simulink model "tune"  (R2018a)
settings: Solver=VariableStepAuto  StartTime=0.0  StopTime=10.0  RelTol=1e-3
libraries: simulink x1, simulink_extras x1
settings Model: Creator=rahul  LastModifiedBy=rahul

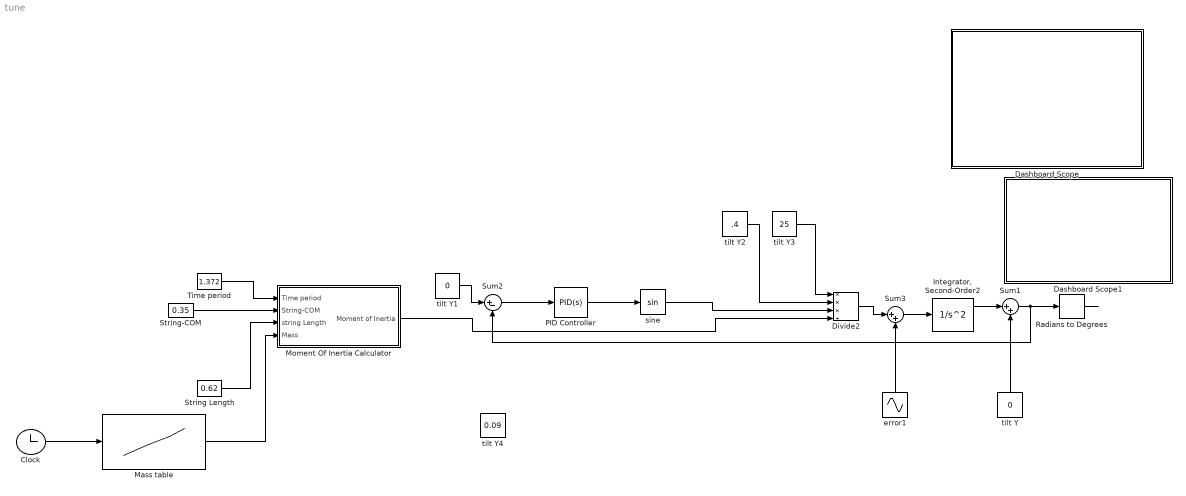
== system tune ==
  Clock : Clock
  Dashboard Scope : Subsystem  DialogController=hmiCreateDDGDialog  IsWebBlock=on  mask(MWDashboardBlock){webBlockId=e338c714-fa8b-4a2a-a1ae-3623556dac48, webBlockType=sdiscope, ShowInitialText=on, HMISrcModelName=tune}
      mask prompts: webBlockId "WebBlock Id"; webBlockType "WebBlock Type"; HMISrcModelName "Source Model"
      mask help: SimulinkHMI:dialogs:HMIScopeDialogDesc
      mask Help: helpview([docroot '/mapfiles/simulink.map'], 'hmi_scope')
      mask Display:
      | if strcmp(get_param(bdroot(gcb),'BlockDiagramType'), 'library')
      |     image([(matlabroot) '/toolbox/simulink/hmi/icons/DashboardScope.png']);
      | end
  Dashboard Scope1 : Subsystem  DialogController=hmiCreateDDGDialog  IsWebBlock=on  mask(MWDashboardBlock){webBlockId=b475c485-489d-4b06-bb0e-a7e4dee8d715, webBlockType=sdiscope, ShowInitialText=on, HMISrcModelName=tune}
      mask prompts: webBlockId "WebBlock Id"; webBlockType "WebBlock Type"; HMISrcModelName "Source Model"
      mask help: SimulinkHMI:dialogs:HMIScopeDialogDesc
      mask Help: helpview([docroot '/mapfiles/simulink.map'], 'hmi_scope')
      mask Display:
      | if strcmp(get_param(bdroot(gcb),'BlockDiagramType'), 'library')
      |     image([(matlabroot) '/toolbox/simulink/hmi/icons/DashboardScope.png']);
      | end
  Divide2 : Product  Inputs=***/
  "Integrator, Second-Order2" : SecondOrderIntegrator
  Mass table : Lookup  InputValues=[0,1]  Table=[0.975,.8]  LookUpMeth=Use Input Nearest  SaturateOnIntegerOverflow=on
  Moment Of Inertia Calculator : Subsystem
  PID Controller : simulink/Continuous/PID Controller  Controller=PID  TimeDomain=Continuous-time  SampleTime=-1  IntegratorMethod=Forward Euler  FilterMethod=Forward Euler  Form=Parallel  UseFilter=on  ControllerParametersSource=internal  P=0.23318201174403  I=0.12576942646477  D=0.085252484006232  N=36.46824066771  InitialConditionSource=internal  InitialConditionForIntegrator=0  InitialConditionForFilter=0  ExternalReset=none  LimitOutput=on  UpperSaturationLimit=0.08726646  LowerSaturationLimit=-0.08726646  LinearizeAsGain=on  AntiWindupMode=none  Kb=1  TrackingMode=off  Kt=1  PParamMin=[]  PParamMax=[]  IParamMin=[]  IParamMax=[]  DParamMin=[]  DParamMax=[]  NParamMin=[]  NParamMax=[]  KbParamMin=[]  KbParamMax=[]  KtParamMin=[]  KtParamMax=[]  POutMin=[]  POutMax=[]  IOutMin=[]  IOutMax=[]  DOutMin=[]  DOutMax=[]  NOutMin=[]  NOutMax=[]  KbOutMin=[]  KbOutMax=[]  KtOutMin=[]  KtOutMax=[]  IntegratorOutMin=[]  IntegratorOutMax=[]  FilterOutMin=[]  FilterOutMax=[]  SumOutMin=[]  SumOutMax=[]  SumI1OutMin=[]  SumI1OutMax=[]  SumI2OutMin=[]  SumI2OutMax=[]  SumI3OutMin=[]  SumI3OutMax=[]  SumDOutMin=[]  SumDOutMax=[]  SaturationOutMin=[]  SaturationOutMax=[]  IntegratorContinuousStateAttributes=''  IntegratorStateMustResolveToSignalObject=off  IntegratorRTWStateStorageClass=Auto  FilterContinuousStateAttributes=''  FilterStateMustResolveToSignalObject=off  FilterRTWStateStorageClass=Auto  DifferentiatorICPrevScaledInput=0  DifferentiatorOutMin=[]  DifferentiatorOutMax=[]  FilterDiffOutCoefMin=[]  FilterDiffOutCoefMax=[]  SumDenOutMin=[]  SumDenOutMax=[]  SumNumOutMin=[]  SumNumOutMax=[]  ReciprocalOutMin=[]  ReciprocalOutMax=[]  DivideOutMin=[]  DivideOutMax=[]  TunerSelectOption=Transfer Function Based (PID Tuner App)
  Radians to Degrees : simulink_extras/Transformations/Radians to Degrees
  String Length : Constant  Value=0.62
  String-COM : Constant  Value=0.35
  Sum1 : Sum  Inputs=|++
  Sum2 : Sum  Inputs=|+-
  Sum3 : Sum  Inputs=|++
  Time period : Constant  Value=1.372
  error1 : Sin  Frequency=4  SampleTime=0
  sine : Trigonometry
  tilt Y : Constant  Value=0
  tilt Y1 : Constant  Value=0
  tilt Y2 : Constant  Value=.4
  tilt Y3 : Constant  Value=25
  tilt Y4 : Constant  Value=0.09
  wires:
  String Length/1 -> Moment Of Inertia Calculator/3(string Length)
  Mass table/1 -> Moment Of Inertia Calculator/4(Mass)
  String-COM/1 -> Moment Of Inertia Calculator/2(String-COM)
  Clock/1 -> Mass table/1
  Time period/1 -> Moment Of Inertia Calculator/1(Time period)
  Sum3/1 -> "Integrator, Second-Order2"/1
  sine/1 -> Divide2/3
  Divide2/1 -> Sum3/1
  "Integrator, Second-Order2"/1 -> Sum1/1
  tilt Y/1 -> Sum1/2
  tilt Y1/1 -> Sum2/1
  tilt Y3/1 -> Divide2/1
  tilt Y2/1 -> Divide2/2
  error1/1 -> Sum3/2
  Moment Of Inertia Calculator/1(Moment of Inertia) -> Divide2/4
  PID Controller/1 -> sine/1
  Sum2/1 -> PID Controller/1
  Sum1/1 -> Radians to Degrees/1, Sum2/2
  Radians to Degrees/1 -> ?

== system tune/Dashboard Scope ==

== system tune/Dashboard Scope1 ==

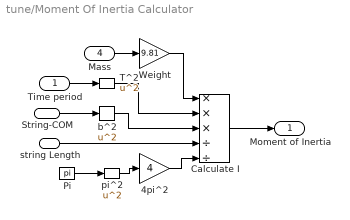
== system tune/Moment Of Inertia Calculator ==
  Time period : Inport
  String-COM : Inport  Port=2
  string Length : Inport  Port=3
  Mass : Inport  Port=4
  4pi^2 : Gain  Gain=4
  Calculate I : Product  Inputs=***//
  Pi : Constant  Value=pi
  T^2 : Math  Operator=square  SaturateOnIntegerOverflow=on
  Weight : Gain  Gain=9.81
  b^2 : Math  Operator=square  SaturateOnIntegerOverflow=on
  pi^2 : Math  Operator=square  SaturateOnIntegerOverflow=on
  Moment of Inertia : Outport
  wires:
  Time period/1 -> T^2/1
  Calculate I/1 -> Moment of Inertia/1
  string Length/1 -> Calculate I/4
  Mass/1 -> Weight/1
  Weight/1 -> Calculate I/1
  pi^2/1 -> 4pi^2/1
  b^2/1 -> Calculate I/3
  T^2/1 -> Calculate I/2
  String-COM/1 -> b^2/1
  Pi/1 -> pi^2/1
  4pi^2/1 -> Calculate I/5
